simulink model "MeanJ2OrbitPropagator"  (R2023a)
settings: Solver=VariableStepAuto  StartTime=0.0  StopTime=10.0  RelTol=1e-3
settings Model: Creator=hugobuurmeijer  LastModifiedBy=hugobuurmeijer

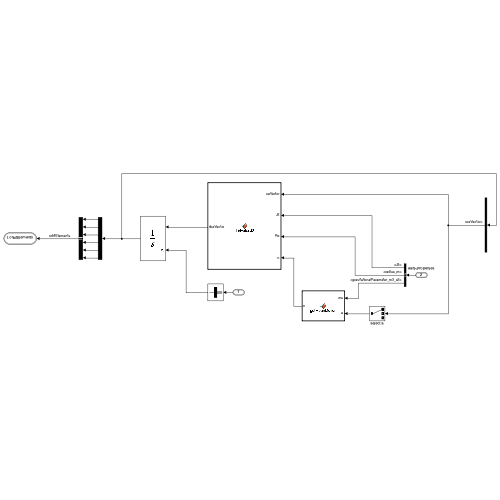
[thumbnail: Simulink's stored preview of the top-level diagram]
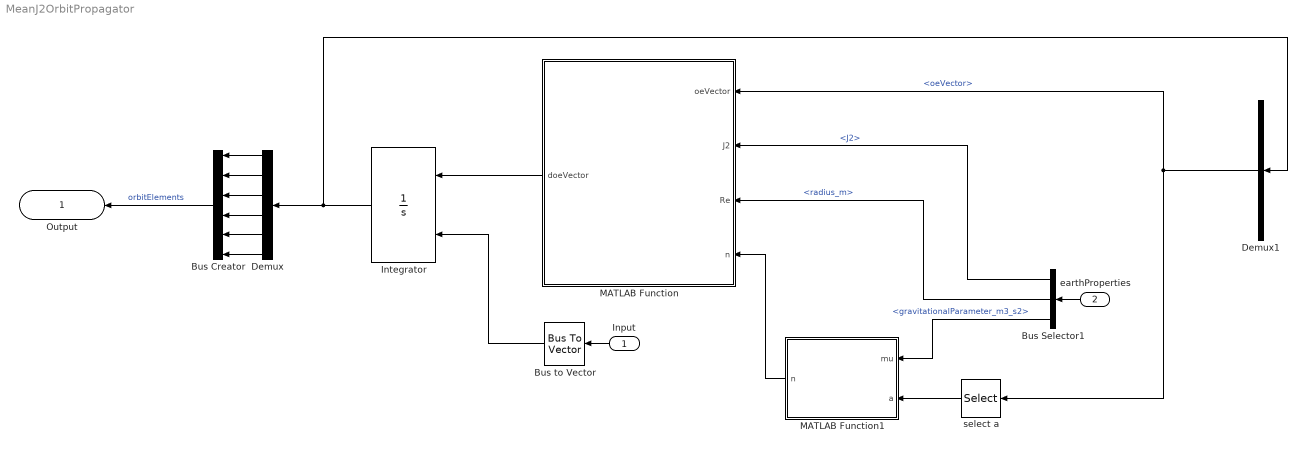
== system MeanJ2OrbitPropagator ==
  Input : Inport  OutDataTypeStr=Bus: orbitElements
  earthProperties : Inport  Port=2  OutDataTypeStr=Bus: earthProperties
  Bus Creator : BusCreator  Inputs=6  OutDataTypeStr=Bus: orbitElements  NonVirtualBus=on
      settings: InheritFromInputs=off
  Bus Selector1 : BusSelector  OutputSignals=J2,radius_m,gravitationalParameter_m3_s2
  Bus to Vector : BusToVector
  Demux : Demux  Outputs=6
  Demux1 : Demux  Outputs=1
  Integrator : Integrator  InitialConditionSource=external
  MATLAB Function : MATLAB Function  TreatAsAtomicUnit=on
  MATLAB Function1 : MATLAB Function  TreatAsAtomicUnit=on
  select a : Selector  InputPortWidth=3  IndexOptions=Index vector (dialog)  Indices=[1]  OutputSizes=1
  Output : Outport  OutDataTypeStr=Bus: orbitElements  BusOutputAsStruct=on
  wires:
  Bus Creator/1 -> Output/1  "orbitElements"
  Demux/6 -> Bus Creator/6
  Demux/2 -> Bus Creator/2
  Demux/3 -> Bus Creator/3
  Bus to Vector/1 -> Integrator/2
  Input/1 -> Bus to Vector/1
  Demux/1 -> Bus Creator/1
  Demux/4 -> Bus Creator/4
  Demux/5 -> Bus Creator/5
  earthProperties/1 -> Bus Selector1/1
  Bus Selector1/1 -> MATLAB Function/2(J2)  "<J2>"
  Bus Selector1/2 -> MATLAB Function/3(Re)  "<radius_m>"
  Bus Selector1/3 -> MATLAB Function1/1(mu)  "<gravitationalParameter_m3_s2>"
  MATLAB Function1/1(n) -> MATLAB Function/4(n)
  Demux1/1 -> MATLAB Function/1(oeVector), select a/1  "<oeVector>"
  select a/1 -> MATLAB Function1/2(a)
  MATLAB Function/1(doeVector) -> Integrator/1
  Integrator/1 -> Demux1/1, Demux/1

== matlab function MeanJ2OrbitPropagator/MATLAB Function1 ==
  data: mu input; a input; n output
function n = getMeanMotion(mu, a)

n = meanMotion(mu, a);

end

== matlab function MeanJ2OrbitPropagator/MATLAB Function ==
  data: oeVector input; J2 input; Re input; n input; doeVector output
function doeVector  = derivatesJ2(oeVector, J2, Re, n)

doeVector = meanDerivatesJ2(oeVector, J2, Re, n);

end
